simulink model "HANcoder_E407_TTA_Group2_REMOTE_72"  (R2018b)
settings: Solver=FixedStepDiscrete  StartTime=0.0  StopTime=1  FixedStep=0.01  RelTol=1e-3
PreLoadFcn:
  | librarySetup
  | eval([bdroot,'_startup']) %Calling [modelName]_startup.m
values from neighbouring files (symbols this model uses):
  BackUp_Role = 4    [HANcoder_E407_TTA_Group2_startup.m]
  basic_cycle_duration_bc0 = TM_Reset_Board   + COMP_duration    (= 320)    [HANcoder_E407_TTA_Group2_startup.m]    (also in HANcoder_E407_TTA_Template_startup.m = 212)
  basic_cycle_duration_bc1 = basic_cycle_duration_bc0    (= 320)    [HANcoder_E407_TTA_Group2_startup.m]    (also in HANcoder_E407_TTA_Template_startup.m = 212)
  board1_online = Simulink.Parameter    [HANcoder_E407_TTA_Group2_startup.m]
  board2_online = Simulink.Parameter    [HANcoder_E407_TTA_Group2_startup.m]
  board3_online = Simulink.Parameter    [HANcoder_E407_TTA_Group2_startup.m]
  board4_online = Simulink.Parameter    [HANcoder_E407_TTA_Group2_startup.m]
  comm_delay_estimation1 = round(comm_delay_measured1*hardware_granularity/frequency_IRQ)    [HANcoder_E407_TTA_Group2_startup.m]    (also in HANcoder_E407_TTA_Template_startup.m)
  comm_delay_estimation2 = round(comm_delay_measured2*hardware_granularity/frequency_IRQ)    [HANcoder_E407_TTA_Group2_startup.m]    (also in HANcoder_E407_TTA_Template_startup.m)
  COMM_Period = 40    [HANcoder_E407_TTA_Group2_startup.m]    (also in HANcoder_E407_TTA_Template_startup.m)
  COMM_Phase1 = Simulink.Parameter    [HANcoder_E407_TTA_Group2_startup.m]    (also in HANcoder_E407_TTA_Template_startup.m)
  COMM_Phase2 = Simulink.Parameter    [HANcoder_E407_TTA_Group2_startup.m]    (also in HANcoder_E407_TTA_Template_startup.m)
  COMM_Phase_init1 = Simulink.Parameter    [HANcoder_E407_TTA_Group2_startup.m]    (also in HANcoder_E407_TTA_Template_startup.m)
  COMM_Phase_init2 = Simulink.Parameter    [HANcoder_E407_TTA_Group2_startup.m]    (also in HANcoder_E407_TTA_Template_startup.m)
  COMP_duration = 8    [HANcoder_E407_TTA_Group2_startup.m]    (also in HANcoder_E407_TTA_Template_startup.m = 4)
  Controller1_Board = 1    [HANcoder_E407_TTA_Group2_startup.m]    (also in HANcoder_E407_TTA_Template_startup.m)
  Controller2_Board = 2    [HANcoder_E407_TTA_Group2_startup.m]    (also in HANcoder_E407_TTA_Template_startup.m)
  Controller3_Board = 3    [HANcoder_E407_TTA_Group2_startup.m]    (also in HANcoder_E407_TTA_Template_startup.m)
  Controller4_Board = 4    [HANcoder_E407_TTA_Group2_startup.m]
  delta_a_set = Simulink.Parameter    [HANcoder_E407_TTA_Group2_startup.m]
  delta_f_set = Simulink.Parameter    [HANcoder_E407_TTA_Group2_startup.m]
  delta_max = 1    [HANcoder_E407_TTA_Group2_startup.m]
  delta_min = -1    [HANcoder_E407_TTA_Group2_startup.m]
  delta_precision = 6    [HANcoder_E407_TTA_Group2_startup.m]
  frequency_IRQ = 100    [HANcoder_E407_TTA_Group2_startup.m]    (also in HANcoder_E407_TTA_Template_startup.m)
  HANtuneOverride = Simulink.Parameter    [HANcoder_E407_TTA_Group2_startup.m]    (also in HANcoder_E407_TTA_Template_startup.m)
  hardware_granularity = 1000000    [HANcoder_E407_TTA_Group2_startup.m]    (also in HANcoder_E407_TTA_Template_startup.m)
  I_a = 2.25    [HANcoder_E407_TTA_Group2_startup.m]
  I_f = 2.25    [HANcoder_E407_TTA_Group2_startup.m]
  idle_time_init = basic_cycle_duration_bc0 + basic_cycle_duration_bc1    (= 640)    [HANcoder_E407_TTA_Group2_startup.m]    (also in HANcoder_E407_TTA_Template_startup.m = 424)
  Input_Gen_Board = 5    [HANcoder_E407_TTA_Group2_startup.m]
  LA_Clock_Gr = 1    [HANcoder_E407_TTA_Group2_startup.m]    (also in HANcoder_E407_TTA_Template_startup.m)
  LA_COMM_dly = 1    [HANcoder_E407_TTA_Group2_startup.m]    (also in HANcoder_E407_TTA_Template_startup.m)
  LA_COMM_Err = 1    [HANcoder_E407_TTA_Group2_startup.m]    (also in HANcoder_E407_TTA_Template_startup.m)
  LA_E_Desync = 1    [HANcoder_E407_TTA_Group2_startup.m]    (also in HANcoder_E407_TTA_Template_startup.m)
  LA_MEX_Flag = 1    [HANcoder_E407_TTA_Group2_startup.m]    (also in HANcoder_E407_TTA_Template_startup.m)
  LA_Task_Act = 1    [HANcoder_E407_TTA_Group2_startup.m]    (also in HANcoder_E407_TTA_Template_startup.m)
  m_v = 100.0    (= 100)    [HANcoder_E407_TTA_Group2_startup.m]
  Master_Role = 1    [HANcoder_E407_TTA_Group2_startup.m]    (also in HANcoder_E407_TTA_Template_startup.m)
  matrix_cycle_duration = basic_cycle_duration_bc0 + basic_cycle_duration_bc1    (= 640)    [HANcoder_E407_TTA_Group2_startup.m]    (also in HANcoder_E407_TTA_Template_startup.m = 424)
  matrix_rows = 2    [HANcoder_E407_TTA_Group2_startup.m]    (also in HANcoder_E407_TTA_Template_startup.m)
  max_desync = 15    [HANcoder_E407_TTA_Group2_startup.m]    (also in HANcoder_E407_TTA_Template_startup.m)
  max_num_msgs_CAN1 = 2^Tx_bit_number-1    (= 7)    [HANcoder_E407_TTA_Group2_startup.m]    (also in HANcoder_E407_TTA_Template_startup.m)
  max_num_msgs_CAN2 = max_num_msgs_CAN1    (= 7)    [HANcoder_E407_TTA_Group2_startup.m]    (also in HANcoder_E407_TTA_Template_startup.m)
  min_desync = (-1)*max_desync    (= -15)    [HANcoder_E407_TTA_Group2_startup.m]    (also in HANcoder_E407_TTA_Template_startup.m)
  OutControl1_ID = 23    [HANcoder_E407_TTA_Group2_startup.m]    (also in HANcoder_E407_TTA_Template_startup.m)
  OutControl2_ID = 24    [HANcoder_E407_TTA_Group2_startup.m]    (also in HANcoder_E407_TTA_Template_startup.m)
  OutEmulator_ID = 25    [HANcoder_E407_TTA_Group2_startup.m]    (also in HANcoder_E407_TTA_Template_startup.m)
  R_al = 0.10    (= 0.1)    [HANcoder_E407_TTA_Group2_startup.m]
  R_ar = 0.10    (= 0.1)    [HANcoder_E407_TTA_Group2_startup.m]
  R_fl = 0.10    (= 0.1)    [HANcoder_E407_TTA_Group2_startup.m]
  R_fr = 0.10    (= 0.1)    [HANcoder_E407_TTA_Group2_startup.m]
  script_run = Simulink.Parameter    [HANcoder_E407_TTA_Group2_startup.m]    (also in HANcoder_E407_TTA_Template_startup.m)
  SensorValues_ID = 22    [HANcoder_E407_TTA_Group2_startup.m]    (also in HANcoder_E407_TTA_Template_startup.m)
  SetValues_ID = 21    [HANcoder_E407_TTA_Group2_startup.m]    (also in HANcoder_E407_TTA_Template_startup.m)
  Slave_Role = 3    [HANcoder_E407_TTA_Group2_startup.m]    (also in HANcoder_E407_TTA_Template_startup.m = 2)
  speed_max = 10    [HANcoder_E407_TTA_Group2_startup.m]
  speed_min = -10    [HANcoder_E407_TTA_Group2_startup.m]
  speed_precision = 3    [HANcoder_E407_TTA_Group2_startup.m]
  Sync_ID = 1    [HANcoder_E407_TTA_Group2_startup.m]    (also in HANcoder_E407_TTA_Template_startup.m)
  tau_max = 5    [HANcoder_E407_TTA_Group2_startup.m]
  tau_min = -5    [HANcoder_E407_TTA_Group2_startup.m]
  testV_1 = Simulink.Parameter    [HANcoder_E407_TTA_Group2_startup.m]
  testV_2 = Simulink.Parameter    [HANcoder_E407_TTA_Group2_startup.m]
  testV_3 = Simulink.Parameter    [HANcoder_E407_TTA_Group2_startup.m]
  theta_max = (speed_max/R_fr)*matrix_cycle_duration*frequency_IRQ/hardware_granularity    (= 6.4)    [HANcoder_E407_TTA_Group2_startup.m]
  theta_min = (-1)*theta_max    (= -6.4)    [HANcoder_E407_TTA_Group2_startup.m]
  theta_precision = 7-(fix(log2(theta_max))+1)    [HANcoder_E407_TTA_Group2_startup.m]
  Tl_a = 0.6    [HANcoder_E407_TTA_Group2_startup.m]
  Tl_f = 0.6    [HANcoder_E407_TTA_Group2_startup.m]
  TM_bc0_1 = basic_cycle_start    (= 0)    [HANcoder_E407_TTA_Group2_startup.m]
  TM_bc0_10 = TM_bc0_9 + COMP_duration    (= 168)    [HANcoder_E407_TTA_Group2_startup.m]
  TM_bc0_11 = TM_bc0_10 + COMP_duration    (= 176)    [HANcoder_E407_TTA_Group2_startup.m]
  TM_bc0_12 = TM_bc0_11  + COMM_duration    (= 216)    [HANcoder_E407_TTA_Group2_startup.m]
  TM_bc0_13 = TM_bc0_12 + COMP_duration    (= 224)    [HANcoder_E407_TTA_Group2_startup.m]
  TM_bc0_14 = TM_bc0_13 + COMP_duration    (= 232)    [HANcoder_E407_TTA_Group2_startup.m]
  TM_bc0_15 = TM_bc0_14  + COMM_duration    (= 272)    [HANcoder_E407_TTA_Group2_startup.m]
  TM_bc0_16 = TM_bc0_15 + COMP_duration    (= 280)    [HANcoder_E407_TTA_Group2_startup.m]
  TM_bc0_17 = TM_bc0_16 + COMP_duration    (= 288)    [HANcoder_E407_TTA_Group2_startup.m]
  TM_bc0_18 = TM_bc0_17 + COMP_duration    (= 296)    [HANcoder_E407_TTA_Group2_startup.m]
  TM_bc0_2 = TM_bc0_1   + COMM_duration    (= 40)    [HANcoder_E407_TTA_Group2_startup.m]
  TM_bc0_3 = TM_bc0_2  + COMP_duration    (= 48)    [HANcoder_E407_TTA_Group2_startup.m]
  TM_bc0_3_2 = TM_bc0_3   + 2    (= 50)    [HANcoder_E407_TTA_Group2_startup.m]
  TM_bc0_4 = TM_bc0_3   + COMP_duration    (= 56)    [HANcoder_E407_TTA_Group2_startup.m]
  TM_bc0_4_2 = TM_bc0_4    + 2    (= 58)    [HANcoder_E407_TTA_Group2_startup.m]
  TM_bc0_5 = TM_bc0_4    + COMP_duration    (= 64)    [HANcoder_E407_TTA_Group2_startup.m]
  TM_bc0_6 = TM_bc0_5  + COMM_duration    (= 104)    [HANcoder_E407_TTA_Group2_startup.m]
  TM_bc0_7 = TM_bc0_6 + COMP_duration    (= 112)    [HANcoder_E407_TTA_Group2_startup.m]
  TM_bc0_8 = TM_bc0_7 + COMP_duration    (= 120)    [HANcoder_E407_TTA_Group2_startup.m]
  TM_bc0_9 = TM_bc0_8  + COMM_duration    (= 160)    [HANcoder_E407_TTA_Group2_startup.m]
  TM_Check_Output_Control1 = TM_COMM_Output_Control1 + COMP_duration    (= 216)    [HANcoder_E407_TTA_Group2_startup.m]
  TM_Check_Sensor_Values = TM_COMM_Sensor_Values + COMM_duration    (= 144)    [HANcoder_E407_TTA_Group2_startup.m]
  TM_Check_Sensor_Values_2 = TM_Check_Sensor_Values + 2    (= 146)    [HANcoder_E407_TTA_Group2_startup.m]
  TM_Check_Set_Values = TM_COMM_Set_Values + COMM_duration    (= 96)    [HANcoder_E407_TTA_Group2_startup.m]
  TM_Check_Set_Values_2 = TM_Check_Set_Values + 2    (= 98)    [HANcoder_E407_TTA_Group2_startup.m]
  TM_Check_Sync = TM_COMM_Sync   + COMM_duration    (= 40)    [HANcoder_E407_TTA_Template_startup.m]
  TM_Check_Vote1 = TM_COMM_Vote1  + COMM_duration    (= 92)    [HANcoder_E407_TTA_Template_startup.m]
  TM_Check_Vote2 = TM_COMM_Vote2  + COMM_duration    (= 140)    [HANcoder_E407_TTA_Template_startup.m]
  TM_Check_Vote2_2 = TM_Check_Vote2 + 2    (= 142)    [HANcoder_E407_TTA_Template_startup.m]
  TM_COMM_Output_Control1 = TM_Velocity + COMM_duration    (= 208)    [HANcoder_E407_TTA_Group2_startup.m]
  TM_COMM_Output_Control1_2 = TM_COMM_Output_Control1 + 2    (= 210)    [HANcoder_E407_TTA_Group2_startup.m]
  TM_COMM_Sensor_Values = TM_Check_Set_Values + COMP_duration    (= 104)    [HANcoder_E407_TTA_Group2_startup.m]
  TM_COMM_Set_Values = TM_bc0_3 + COMP_duration    (= 56)    [HANcoder_E407_TTA_Group2_startup.m]
  TM_COMM_Sync = basic_cycle_start    (= 0)    [HANcoder_E407_TTA_Group2_startup.m]    (also in HANcoder_E407_TTA_Template_startup.m)
  TM_Count_Vote1 = TM_Check_Vote1 + COMP_duration    (= 96)    [HANcoder_E407_TTA_Template_startup.m]
  TM_Data_bc0 = TM_COMM_Sync    (= 0)    [HANcoder_E407_TTA_Group2_startup.m]    (also in HANcoder_E407_TTA_Template_startup.m)
  TM_Data_bc1 = TM_Data_bc0(1:4)    [HANcoder_E407_TTA_Group2_startup.m]    (also in HANcoder_E407_TTA_Template_startup.m)
  TM_Reset_Board = TM_Reset_Var   + COMP_duration    (= 312)    [HANcoder_E407_TTA_Group2_startup.m]    (also in HANcoder_E407_TTA_Template_startup.m = 208)
  TM_Reset_Var = TM_bc0_18  + COMP_duration    (= 304)    [HANcoder_E407_TTA_Group2_startup.m]    (also in HANcoder_E407_TTA_Template_startup.m = 204)
  TM_Reset_Var_bc1 = TM_bc0_14 + COMP_duration    (= 240)    [HANcoder_E407_TTA_Group2_startup.m]    (also in HANcoder_E407_TTA_Template_startup.m = 200)
  TM_Reset_Var_bc1_2 = TM_Reset_Var_bc1 + 2    (= 242)    [HANcoder_E407_TTA_Group2_startup.m]    (also in HANcoder_E407_TTA_Template_startup.m = 202)
  TM_Steer = TM_Check_Sensor_Values + COMP_duration    (= 152)    [HANcoder_E407_TTA_Group2_startup.m]
  TM_Torque = TM_Steer + COMP_duration    (= 160)    [HANcoder_E407_TTA_Group2_startup.m]
  TM_Type_bc0 = COMM    (= 0)    [HANcoder_E407_TTA_Group2_startup.m]    (also in HANcoder_E407_TTA_Template_startup.m)
  TM_Type_bc1 = TM_Type_bc0(1:4)    [HANcoder_E407_TTA_Group2_startup.m]    (also in HANcoder_E407_TTA_Template_startup.m)
  TM_Update_LT = TM_Check_Sync  + COMP_duration    (= 44)    [HANcoder_E407_TTA_Template_startup.m]
  TM_Update_LT_2 = TM_Update_LT   + 2    (= 46)    [HANcoder_E407_TTA_Template_startup.m]
  TM_Velocity = TM_Torque + COMP_duration    (= 168)    [HANcoder_E407_TTA_Group2_startup.m]
  TM_Vote_Dec = TM_Update_LT   + COMP_duration    (= 48)    [HANcoder_E407_TTA_Template_startup.m]
  torque_precision = 4    [HANcoder_E407_TTA_Group2_startup.m]
  ... (+7 more)
undefined symbols (not defined in the file or in its folder): A0, A1, A2, A3, A4, CON2, CON4, D10, D12, D13, D8, D9, TM_Check_Output_Emulator, TM_Check_Output_Emulator_2, TM_COMM_Output_Emulator
libraries: hdlsllib x247, HANcoder_STM32_Target x28, simulink x5, simulink_extras x1
(part 7 of 29)

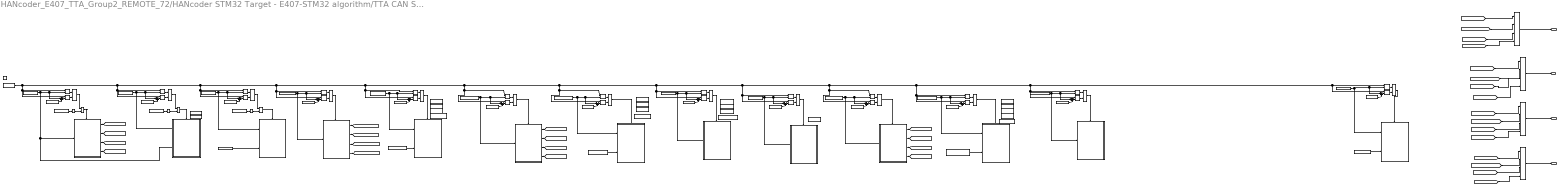
== system HANcoder_E407_TTA_Group2_REMOTE_72/HANcoder STM32 Target - E407-STM32 algorithm/TTA CAN System/TTA System/Matrix Cycle Manager/Controller Matrix Cycle/controller basic cycle 1 ==
  note: Output Send_Message
      | Send: 1
      | Do not send: 0
  note: Output Receive_Message
      | Receive: 1
      | Do not receive: 0
  note: Output Receive_Message
      | Receive: 1
      | Do not receive: 0
  note: Output Send_Message
      | Send: 1
      | Do not send: 0
  note: COMM - TW check
  note: COMP - TW check
  note: Local Time still not updated
  note: COMP - TW check
  note: Local Time still not updated
  note: Local Time still not updated
  note: COMP - TW check
  note: COMM - TW check
  note: COMP - TW check
  note: Send message condition
      | Sync Msg: Master and TM0
      | Vote Msg: Node# and TM#
  note: COMP - TW check
  note: COMP - TW check
  note: COMP - TW check
  note: COMM - TW check
  note: COMM - TW check
  note: COMP - TW check
  note: COMP - TW check
  Enable : EnablePort
  AND{,1..11,17..20} (16 alike) : Logic  IconShape=distinctive  AllPortsSameDT=off  OutDataTypeStr=boolean
  COMM Task - Set_Values : Subsystem
  COMM Task - Sync bc 1 : Subsystem
  COMM Task - Test1 : Subsystem
  COMM Task - send_BS : Subsystem
  "COMP Task - Do calculations " : Subsystem
  COMP Task - Get master Up to date : Subsystem
  COMP Task - Process_BS_Msg : Subsystem
  COMP Task - Reset Variables BC1 : Subsystem
  COMP Task - Rx_Set_Values_Check : Subsystem
  COMP Task - Sync bc1 check : Subsystem
  COMP Task - Test Receive1 : Subsystem
  COMP Task - Update LT1 : Subsystem
  COMP Task - Voting : Subsystem
  Constant : Constant  Value=TM_bc0_1
  Constant{1,10,18,21} (4 alike) : Constant  Value=COMM_Period
  Constant{2..3,9,11,15,20,22,27,29} (9 alike) : Constant  Value=COMP_duration
  Constant12 : Constant  Value=TM_COMM_Output_Control1
  Constant13 : Constant  Value=TM_COMM_Output_Control1_2
  Constant14 : Constant  Value=TM_Torque
  Constant16 : Constant  Value=TM_Reset_Var_bc1
  Constant17 : Constant  Value=TM_bc0_3_2
  Constant19 : Constant  Value=TM_Check_Set_Values_2
  Constant23 : Constant  Value=TM_Check_Sensor_Values
  Constant24 : Constant  Value=TM_Check_Sensor_Values_2
  Constant25 : Constant  Value=TM_COMM_Sensor_Values
  Constant26 : Constant  Value=TM_Check_Output_Control1
  Constant28 : Constant  Value=TM_Steer
  Constant4 : Constant  Value=TM_bc0_2
  Constant41 : Constant  Value=TM_Reset_Var_bc1_2
  Constant5 : Constant  Value=TM_COMM_Set_Values
  Constant6 : Constant  Value=TM_bc0_3
  Constant7 : Constant  Value=TM_Check_Set_Values
  Constant8 : Constant  Value=TM_Velocity
  Data Store Memory1 : DataStoreMemory  DataStoreName=Error_BS_NotRX  ReadBeforeWriteMsg=warning  WriteAfterWriteMsg=warning  WriteAfterReadMsg=warning  ShowAdditionalParam=off  OutDataTypeStr=boolean
  Data Store Memory10 : DataStoreMemory  DataStoreName=v_set_stored  ReadBeforeWriteMsg=warning  WriteAfterWriteMsg=warning  WriteAfterReadMsg=warning  ShowAdditionalParam=off
  Data Store Memory11 : DataStoreMemory  DataStoreName=Msg_Rx  ReadBeforeWriteMsg=warning  WriteAfterWriteMsg=warning  WriteAfterReadMsg=warning  ShowAdditionalParam=off  OutDataTypeStr=Bus: msg_buffer_type
  Data Store Memory12 : DataStoreMemory  DataStoreName=Error_SensorValues_NotRX  ReadBeforeWriteMsg=warning  WriteAfterWriteMsg=warning  WriteAfterReadMsg=warning  ShowAdditionalParam=off  OutDataTypeStr=boolean
  Data Store Memory13 : DataStoreMemory  DataStoreName=Error_Test_NotRX  ReadBeforeWriteMsg=warning  WriteAfterWriteMsg=warning  WriteAfterReadMsg=warning  ShowAdditionalParam=off  OutDataTypeStr=boolean
  Data Store Memory14 : DataStoreMemory  DataStoreName=rxTest3  ReadBeforeWriteMsg=warning  WriteAfterWriteMsg=warning  WriteAfterReadMsg=warning  ShowAdditionalParam=off
  Data Store Memory15 : DataStoreMemory  DataStoreName=rxTest1  ReadBeforeWriteMsg=warning  WriteAfterWriteMsg=warning  WriteAfterReadMsg=warning  ShowAdditionalParam=off
  Data Store Memory16 : DataStoreMemory  DataStoreName=rxTest2  ReadBeforeWriteMsg=warning  WriteAfterWriteMsg=warning  WriteAfterReadMsg=warning  ShowAdditionalParam=off
  Data Store Memory17 : DataStoreMemory  DataStoreName=B2  ReadBeforeWriteMsg=warning  WriteAfterWriteMsg=warning  WriteAfterReadMsg=warning  ShowAdditionalParam=off
  Data Store Memory2 : DataStoreMemory  DataStoreName=B4  ReadBeforeWriteMsg=warning  WriteAfterWriteMsg=warning  WriteAfterReadMsg=warning  ShowAdditionalParam=off
  Data Store Memory20 : DataStoreMemory  DataStoreName=delta_f_set_stored  ReadBeforeWriteMsg=warning  WriteAfterWriteMsg=warning  WriteAfterReadMsg=warning  ShowAdditionalParam=off
  Data Store Memory28 : DataStoreMemory  DataStoreName=Error_SetValues_NotRX  ReadBeforeWriteMsg=warning  WriteAfterWriteMsg=warning  WriteAfterReadMsg=warning  ShowAdditionalParam=off  OutDataTypeStr=boolean
  Data Store Memory3 : DataStoreMemory  DataStoreName=B3  ReadBeforeWriteMsg=warning  WriteAfterWriteMsg=warning  WriteAfterReadMsg=warning  ShowAdditionalParam=off
  Data Store Memory31 : DataStoreMemory  DataStoreName=delta_a_set_stored  ReadBeforeWriteMsg=warning  WriteAfterWriteMsg=warning  WriteAfterReadMsg=warning  ShowAdditionalParam=off
  Data Store Memory4 : DataStoreMemory  DataStoreName=B1  ReadBeforeWriteMsg=warning  WriteAfterWriteMsg=warning  WriteAfterReadMsg=warning  ShowAdditionalParam=off
  Data Store Memory5 : DataStoreMemory  DataStoreName=Test3  ReadBeforeWriteMsg=warning  WriteAfterWriteMsg=warning  WriteAfterReadMsg=warning  ShowAdditionalParam=off
  Data Store Memory6 : DataStoreMemory  DataStoreName=Test1  ReadBeforeWriteMsg=warning  WriteAfterWriteMsg=warning  WriteAfterReadMsg=warning  ShowAdditionalParam=off
  Data Store Memory7 : DataStoreMemory  DataStoreName=Test2  ReadBeforeWriteMsg=warning  WriteAfterWriteMsg=warning  WriteAfterReadMsg=warning  ShowAdditionalParam=off
  Data Store Memory8 : DataStoreMemory  DataStoreName=new_msg_Rx  ReadBeforeWriteMsg=warning  WriteAfterWriteMsg=warning  WriteAfterReadMsg=warning  ShowAdditionalParam=off
  Data Store Memory9 : DataStoreMemory  DataStoreName=votingOut  ReadBeforeWriteMsg=warning  WriteAfterWriteMsg=warning  WriteAfterReadMsg=warning  ShowAdditionalParam=off
  Data Store Read1 : DataStoreRead  DataStoreName=Local_Ticks
  Data Store Read11 : DataStoreRead  DataStoreName=BC1_Sync_processed
  Data Store Read6 : DataStoreRead  DataStoreName=BC1_Sync_processed
  Data Store Read7 : DataStoreRead  DataStoreName=BC1_Sync_processed
  GreaterThan{,2,4,6,8,10,12,14,16,18,20,22,34} (13 alike) : RelationalOperator  OutDataTypeStr=boolean  RndMeth=Simplest
  GreaterThan{1,3,5,7,9,11,13,15,17,19,21,23,35} (13 alike) : RelationalOperator  Operator=<  OutDataTypeStr=boolean  RndMeth=Simplest
  NOT2 : Logic  Operator=NOT  IconShape=distinctive  AllPortsSameDT=off  OutDataTypeStr=boolean
  NOT4 : Logic  Operator=NOT  IconShape=distinctive  AllPortsSameDT=off  OutDataTypeStr=boolean
  NOT5 : Logic  Operator=NOT  IconShape=distinctive  AllPortsSameDT=off  OutDataTypeStr=boolean
  OR{1..4} (4 alike) : Logic  Operator=OR  Inputs=4  IconShape=distinctive  AllPortsSameDT=off  OutDataTypeStr=boolean
  Sum{1..12,18} (13 alike) : Sum  Inputs=|++
  Send_Message_CAN1 : Outport  OutputWhenDisabled=reset  InitialOutput=0
  Send_Message_CAN2 : Outport  Port=2  OutputWhenDisabled=reset  InitialOutput=0
  Receive_Message_CAN1 : Outport  Port=3  OutputWhenDisabled=reset  InitialOutput=0
  Receive_Message_CAN2 : Outport  Port=4  OutputWhenDisabled=reset  InitialOutput=0
  wires:
  Constant1/1 -> Sum4/2
  COMM Task - Sync bc 1/1(Send CAN1) -> [send_CAN1_Sync_bc1_TAG]
  COMM Task - Sync bc 1/2(Receive CAN1) -> [receive_CAN1_Sync_bc1_TAG]
  COMM Task - Sync bc 1/4(Receive CAN2) -> [receive_CAN2_Sync_bc1_TAG]
  AND19/1 -> COMP Task - Update LT1/Enable
  NOT2/1 -> AND18/2
  Data Store Read7/1 -> NOT5/1
  GreaterThan4/1 -> AND2/1
  AND18/1 -> COMP Task - Sync bc1 check/Enable
  AND1/1 -> AND18/1
  Data Store Read11/1 -> NOT4/1
  AND17/1 -> COMM Task - Sync bc 1/Enable
  AND2/1 -> AND19/1
  Data Store Read6/1 -> NOT2/1
  NOT4/1 -> AND17/2
  GreaterThan1/1 -> AND/2
  GreaterThan/1 -> AND/1
  Constant/1 -> COMP Task - Sync bc1 check/2(TM_COMM), COMM Task - Sync bc 1/1(Time Mark), Sum4/1, GreaterThan/2
  AND/1 -> AND17/1
  Constant3/1 -> Sum2/2
  Constant6/1 -> COMP Task - Update LT1/1(Time_Mark), Sum2/1, GreaterThan4/2
  Sum4/1 -> GreaterThan1/2
  GreaterThan2/1 -> AND1/1
  GreaterThan3/1 -> AND1/2
  Constant2/1 -> Sum1/2
  Constant4/1 -> COMP Task - Sync bc1 check/1(Time_Mark), GreaterThan2/2, Sum1/1
  Sum1/1 -> GreaterThan3/2
  COMM Task - Sync bc 1/3(Send CAN2) -> [send_CAN2_Sync_bc1_TAG]
  NOT5/1 -> AND19/2
  Sum2/1 -> GreaterThan5/2
  GreaterThan5/1 -> AND2/2
  GreaterThan35/1 -> AND20/2
  Constant16/1 -> Sum18/1, GreaterThan34/2, COMP Task - Reset Variables BC1/1(Time_Mark)
  Constant15/1 -> Sum18/2
  Sum18/1 -> GreaterThan35/2
  GreaterThan34/1 -> AND20/1
  AND20/1 -> COMP Task - Reset Variables BC1/Enable
  Constant17/1 -> COMP Task - Update LT1/2(Time_Mark_2)
  Constant41/1 -> COMP Task - Reset Variables BC1/2(Time_Mark_2)
  GreaterThan7/1 -> AND3/2
  COMM Task - Set_Values/2(Receive CAN1) -> [receive_CAN1_Set_Values_bc1_TAG]
  Sum5/1 -> GreaterThan9/2
  COMM Task - Set_Values/4(Receive CAN2) -> [receive_CAN2_Set_Values_bc1_TAG]
  COMM Task - Set_Values/3(Send CAN2) -> [send_CAN2_Set_Values_bc1_TAG]
  GreaterThan6/1 -> AND3/1
  COMM Task - Set_Values/1(Send CAN1) -> [send_CAN1_Set_Values_bc1_TAG]
  Constant19/1 -> COMP Task - Rx_Set_Values_Check/2(Time_Mark_2)
  GreaterThan9/1 -> AND4/2
  AND4/1 -> COMP Task - Rx_Set_Values_Check/Enable
  GreaterThan8/1 -> AND4/1
  Constant9/1 -> Sum5/2
  Sum3/1 -> GreaterThan7/2
  Constant7/1 -> COMP Task - Rx_Set_Values_Check/1(Time_Mark), Sum5/1, GreaterThan8/2
  Constant18/1 -> Sum3/2
  Constant5/1 -> COMM Task - Set_Values/1(Time Mark), GreaterThan6/2, Sum3/1
  AND3/1 -> COMM Task - Set_Values/Enable
  OR1/1 -> Send_Message_CAN1/1
  [send_CAN1_Set_Values_bc1_TAG] -> OR1/2
  [send_CAN1_Sync_bc1_TAG] -> OR1/1
  [receive_CAN2_Sync_bc1_TAG] -> OR4/1
  [receive_CAN1_Sync_bc1_TAG] -> OR3/1
  [send_CAN2_Sync_bc1_TAG] -> OR2/1
  OR3/1 -> Receive_Message_CAN1/1
  OR4/1 -> Receive_Message_CAN2/1
  [send_CAN2_Set_Values_bc1_TAG] -> OR2/2
  [receive_CAN1_Set_Values_bc1_TAG] -> OR3/2
  [receive_CAN2_Set_Values_bc1_TAG] -> OR4/2
  OR2/1 -> Send_Message_CAN2/1
  [receive_CAN2_Test_bc1_TAG] -> OR4/3
  [receive_CAN1_Test_bc1_TAG] -> OR3/3
  [send_CAN2_Test_bc1_TAG] -> OR2/3
  [send_CAN1_Test_bc1_TAG] -> OR1/3
  Constant29/1 -> Sum8/2
  Sum8/1 -> GreaterThan19/2
  GreaterThan18/1 -> AND7/1
  GreaterThan19/1 -> AND7/2
  AND7/1 -> "COMP Task - Do calculations "/Enable
  Constant28/1 -> "COMP Task - Do calculations "/1(Time_Mark), GreaterThan18/2, Sum8/1
  Constant14/1 -> COMP Task - Voting/1(Time_Mark), GreaterThan14/2, Sum9/1
  GreaterThan15/1 -> AND8/2
  Constant20/1 -> Sum9/2
  AND8/1 -> COMP Task - Voting/Enable
  GreaterThan14/1 -> AND8/1
  Sum9/1 -> GreaterThan15/2
  GreaterThan17/1 -> AND9/2
  AND10/1 -> COMP Task - Test Receive1/Enable
  COMM Task - Test1/3(Send CAN2) -> [send_CAN2_Test_bc1_TAG]
  GreaterThan21/1 -> AND10/2
  Constant22/1 -> Sum10/2
  Constant25/1 -> COMM Task - Test1/1(Time Mark), Sum11/1, GreaterThan16/2
  GreaterThan16/1 -> AND9/1
  Constant21/1 -> Sum11/2
  Sum11/1 -> GreaterThan17/2
  AND9/1 -> COMM Task - Test1/Enable
  Sum10/1 -> GreaterThan21/2
  COMM Task - Test1/4(Receive CAN2) -> [receive_CAN2_Test_bc1_TAG]
  Constant23/1 -> COMP Task - Test Receive1/1(Time_Mark), GreaterThan20/2, Sum10/1
  GreaterThan20/1 -> AND10/1
  Constant24/1 -> COMP Task - Test Receive1/2(Time_Mark_2)
  COMM Task - Test1/2(Receive CAN1) -> [receive_CAN1_Test_bc1_TAG]
  COMM Task - Test1/1(Send CAN1) -> [send_CAN1_Test_bc1_TAG]
  Constant11/1 -> Sum6/2
  Sum7/1 -> GreaterThan11/2
  Constant13/1 -> COMP Task - Process_BS_Msg/2(Time_Mark_2)
  Constant10/1 -> Sum7/2
  AND5/1 -> COMM Task - send_BS/Enable
  Constant8/1 -> COMM Task - send_BS/1(Time Mark), Sum7/1, GreaterThan10/2
  Constant12/1 -> COMP Task - Process_BS_Msg/1(Time_Mark), GreaterThan12/2, Sum6/1
  COMM Task - send_BS/4(Receive CAN2) -> [receive_CAN2_BS_bc1_TAG]
  Sum6/1 -> GreaterThan13/2
  GreaterThan12/1 -> AND6/1
  COMM Task - send_BS/2(Receive CAN1) -> [receive_CAN1_BS_bc1_TAG]
  COMM Task - send_BS/1(Send CAN1) -> [send_CAN1_BS_bc1_TAG]
  GreaterThan13/1 -> AND6/2
  AND6/1 -> COMP Task - Process_BS_Msg/Enable
  GreaterThan11/1 -> AND5/2
  COMM Task - send_BS/3(Send CAN2) -> [send_CAN2_BS_bc1_TAG]
  GreaterThan10/1 -> AND5/1
  [send_CAN1_BS_bc1_TAG] -> OR1/4
  [send_CAN2_BS_bc1_TAG] -> OR2/4
  [receive_CAN2_BS_bc1_TAG] -> OR4/4
  [receive_CAN1_BS_bc1_TAG] -> OR3/4
  Constant27/1 -> Sum12/2
  GreaterThan22/1 -> AND11/1
  Constant26/1 -> COMP Task - Get master Up to date/1(Time_Mark), GreaterThan22/2, Sum12/1
  Sum12/1 -> GreaterThan23/2
  AND11/1 -> COMP Task - Get master Up to date/Enable
  GreaterThan23/1 -> AND11/2
  Data Store Read1/1 -> GreaterThan7/1, GreaterThan6/1, GreaterThan17/1, GreaterThan16/1, GreaterThan21/1, GreaterThan20/1, GreaterThan14/1, GreaterThan15/1, GreaterThan11/1, GreaterThan10/1, GreaterThan12/1, GreaterThan13/1, GreaterThan22/1, GreaterThan23/1, GreaterThan34/1, GreaterThan35/1, GreaterThan18/1, GreaterThan19/1, GreaterThan8/1, GreaterThan9/1, GreaterThan4/1, GreaterThan5/1, GreaterThan2/1, GreaterThan3/1, GreaterThan/1, GreaterThan1/1

== system HANcoder_E407_TTA_Group2_REMOTE_72/HANcoder STM32 Target - E407-STM32 algorithm/TTA CAN System/TTA System/Matrix Cycle Manager/Controller Matrix Cycle/msg_count_DEBUG observer ==
  Data Store Read24 : DataStoreRead  DataStoreName=msg_count_DEBUG
  Terminator : Terminator
  wires:
  Data Store Read24/1 -> Terminator/1  "msg_count_DEBUG_s"

== system HANcoder_E407_TTA_Group2_REMOTE_72/HANcoder STM32 Target - E407-STM32 algorithm/TTA CAN System/TTA System/Matrix Cycle Manager/Input Generator Matrix Cycle/Matrix_Cycle_Observation_DEBUG ==
  Data Store Read : DataStoreRead  DataStoreName=Master_ID
  Data Store Read1 : DataStoreRead  DataStoreName=Role_ID
  Data Store Read10 : DataStoreRead  DataStoreName=BC1_Sync_processed
  Data Store Read2 : DataStoreRead  DataStoreName=BC0_Sync_processed
  Data Store Read3 : DataStoreRead  DataStoreName=Sync_bc1_missed_counter
  Data Store Read4 : DataStoreRead  DataStoreName=Sync_bc0_missed_counter
  Terminator{,1..4,12} (6 alike) : Terminator
  wires:
  Data Store Read1/1 -> Terminator/1  "Role_ID_ing_s"
  Data Store Read10/1 -> Terminator12/1  "BC1_sync_processed_ing_s"
  Data Store Read2/1 -> Terminator2/1  "BC0_sync_processed_ing_s"
  Data Store Read/1 -> Terminator1/1  "Master_ID_ing_s"
  Data Store Read3/1 -> Terminator4/1  "sync_bc1_miss_counter_ing"
  Data Store Read4/1 -> Terminator3/1  "sync_bc0_miss_counter_ing"

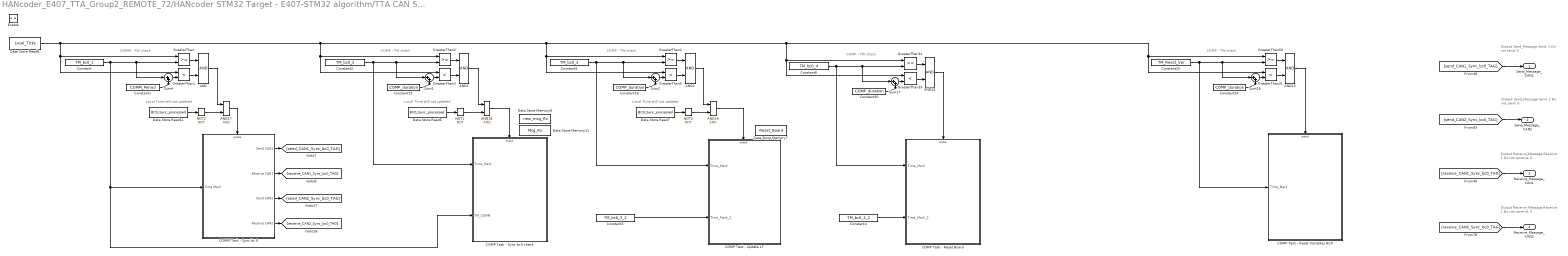
== system HANcoder_E407_TTA_Group2_REMOTE_72/HANcoder STM32 Target - E407-STM32 algorithm/TTA CAN System/TTA System/Matrix Cycle Manager/Input Generator Matrix Cycle/input generator basic cycle 0 ==
  note: Local Time still not updated
  note: Local Time still not updated
  note: Local Time still not updated
  note: COMP - TW check
  note: COMP - TW check
  note: COMP - TW check
  note: COMP - TW check
  note: COMM - TW check
  note: Output Receive_Message
      | Receive: 1
      | Do not receive: 0
  note: Output Send_Message
      | Send: 1
      | Do not send: 0
  note: Output Receive_Message
      | Receive: 1
      | Do not receive: 0
  note: Output Send_Message
      | Send: 1
      | Do not send: 0
  Enable : EnablePort  PropagateVarSize=During execution
  AND{,1..2,15..19} (8 alike) : Logic  IconShape=distinctive  AllPortsSameDT=off  OutDataTypeStr=boolean
  COMM Task - Sync bc 0 : Subsystem
  COMP Task - Reset Board : Subsystem
  COMP Task - Reset Variables BC0 : Subsystem
  COMP Task - Sync bc0 check : Subsystem
  COMP Task - Update LT : Subsystem
  Constant : Constant  Value=TM_bc0_1
  Constant1 : Constant  Value=COMM_Period
  Constant{15..16,24,30} (4 alike) : Constant  Value=COMP_duration
  Constant2 : Constant  Value=TM_bc0_2
  Constant25 : Constant  Value=TM_Reset_Var
  Constant3 : Constant  Value=TM_bc0_3_2
  Constant4 : Constant  Value=TM_bc0_4_2
  Constant5 : Constant  Value=TM_bc0_3
  Constant6 : Constant  Value=TM_bc0_4
  Data Store Memory11 : DataStoreMemory  DataStoreName=Msg_Rx  ReadBeforeWriteMsg=warning  WriteAfterWriteMsg=warning  WriteAfterReadMsg=warning  ShowAdditionalParam=off  OutDataTypeStr=Bus: msg_buffer_type
  Data Store Memory7 : DataStoreMemory  DataStoreName=Reset_Board  ReadBeforeWriteMsg=warning  WriteAfterWriteMsg=warning  WriteAfterReadMsg=warning  ShowAdditionalParam=off  OutDataTypeStr=boolean
  Data Store Memory8 : DataStoreMemory  DataStoreName=new_msg_Rx  ReadBeforeWriteMsg=warning  WriteAfterWriteMsg=warning  WriteAfterReadMsg=warning  ShowAdditionalParam=off
  Data Store Read11 : DataStoreRead  DataStoreName=BC0_Sync_processed
  Data Store Read6 : DataStoreRead  DataStoreName=BC0_Sync_processed
  Data Store Read7 : DataStoreRead  DataStoreName=BC0_Sync_processed
  Data Store Read8 : DataStoreRead  DataStoreName=Local_Ticks
  GreaterThan{,2,4,30,32} (5 alike) : RelationalOperator  OutDataTypeStr=boolean  RndMeth=Simplest
  GreaterThan{1,3,5,31,33} (5 alike) : RelationalOperator  Operator=<  OutDataTypeStr=boolean  RndMeth=Simplest
  NOT1 : Logic  Operator=NOT  IconShape=distinctive  AllPortsSameDT=off  OutDataTypeStr=boolean
  NOT2 : Logic  Operator=NOT  IconShape=distinctive  AllPortsSameDT=off  OutDataTypeStr=boolean
  NOT3 : Logic  Operator=NOT  IconShape=distinctive  AllPortsSameDT=off  OutDataTypeStr=boolean
  Sum{1..2,4,16..17} (5 alike) : Sum  Inputs=|++
  Send_Message_CAN1 : Outport  OutputWhenDisabled=reset  InitialOutput=0
  Send_Message_CAN2 : Outport  Port=2  OutputWhenDisabled=reset  InitialOutput=0
  Receive_Message_CAN1 : Outport  Port=3  OutputWhenDisabled=reset  InitialOutput=0
  Receive_Message_CAN2 : Outport  Port=4  OutputWhenDisabled=reset  InitialOutput=0
  wires:
  AND19/1 -> COMP Task - Update LT/Enable
  AND2/1 -> AND19/1
  NOT3/1 -> AND19/2
  Data Store Read7/1 -> NOT3/1
  AND18/1 -> COMP Task - Sync bc0 check/Enable
  AND1/1 -> AND18/1
  NOT1/1 -> AND18/2
  Data Store Read6/1 -> NOT1/1
  AND17/1 -> COMM Task - Sync bc 0/Enable
  NOT2/1 -> AND17/2
  Data Store Read11/1 -> NOT2/1
  GreaterThan33/1 -> AND16/2
  Sum17/1 -> GreaterThan33/2
  GreaterThan32/1 -> AND16/1
  Constant30/1 -> Sum17/2
  Constant6/1 -> GreaterThan32/2, Sum17/1, COMP Task - Reset Board/1(Time_Mark)
  AND16/1 -> COMP Task - Reset Board/Enable
  Data Store Read8/1 -> GreaterThan1/1, GreaterThan/1, GreaterThan3/1, GreaterThan2/1, GreaterThan5/1, GreaterThan4/1, GreaterThan30/1, GreaterThan31/1, GreaterThan33/1, GreaterThan32/1
  AND15/1 -> COMP Task - Reset Variables BC0/Enable
  Constant25/1 -> Sum16/1, GreaterThan30/2, COMP Task - Reset Variables BC0/1(Time_Mark)
  Constant24/1 -> Sum16/2
  GreaterThan30/1 -> AND15/1
  Sum16/1 -> GreaterThan31/2
  GreaterThan31/1 -> AND15/2
  GreaterThan5/1 -> AND2/2
  GreaterThan4/1 -> AND2/1
  Sum2/1 -> GreaterThan5/2
  Constant5/1 -> GreaterThan4/2, Sum2/1, COMP Task - Update LT/1(Time_Mark)
  Constant16/1 -> Sum2/2
  Constant15/1 -> Sum1/2
  Constant2/1 -> Sum1/1, GreaterThan2/2, COMP Task - Sync bc0 check/1(Time_Mark)
  Sum1/1 -> GreaterThan3/2
  GreaterThan2/1 -> AND1/1
  GreaterThan3/1 -> AND1/2
  AND/1 -> AND17/1
  GreaterThan1/1 -> AND/2
  GreaterThan/1 -> AND/1
  Sum4/1 -> GreaterThan1/2
  Constant/1 -> GreaterThan/2, Sum4/1, COMM Task - Sync bc 0/1(Time Mark), COMP Task - Sync bc0 check/2(TM_COMM)
  Constant1/1 -> Sum4/2
  COMM Task - Sync bc 0/4(Receive CAN2) -> [receive_CAN2_Sync_bc0_TAG]
  COMM Task - Sync bc 0/3(Send CAN2) -> [send_CAN2_Sync_bc0_TAG]
  COMM Task - Sync bc 0/2(Receive CAN1) -> [receive_CAN1_Sync_bc0_TAG]
  COMM Task - Sync bc 0/1(Send CAN1) -> [send_CAN1_Sync_bc0_TAG]
  [send_CAN1_Sync_bc0_TAG] -> Send_Message_CAN1/1
  [send_CAN2_Sync_bc0_TAG] -> Send_Message_CAN2/1
  [receive_CAN1_Sync_bc0_TAG] -> Receive_Message_CAN1/1
  [receive_CAN2_Sync_bc0_TAG] -> Receive_Message_CAN2/1
  Constant3/1 -> COMP Task - Update LT/2(Time_Mark_2)
  Constant4/1 -> COMP Task - Reset Board/2(Time_Mark_2)

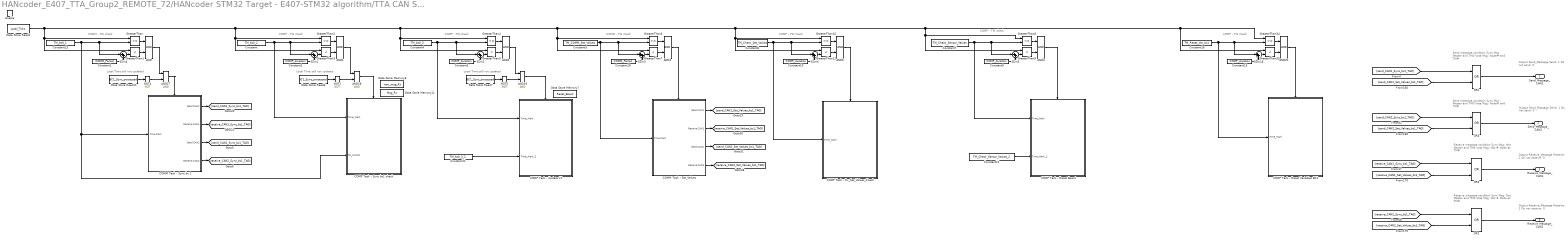
== system HANcoder_E407_TTA_Group2_REMOTE_72/HANcoder STM32 Target - E407-STM32 algorithm/TTA CAN System/TTA System/Matrix Cycle Manager/Input Generator Matrix Cycle/input generator basic cycle 1 ==
  note: COMP - TW check
  note: COMM - TW check
  note: Local Time still not updated
  note: Local Time still not updated
  note: COMP - TW check
  note: Local Time still not updated
  note: COMP - TW check
  note: COMP - TW check
  note: COMM - TW check
  note: Receive message condition
      | Sync Msg: Not Master and TM0
      | Vote Msg: Not # Node at TM#
  note: Send message condition
      | Sync Msg: Master and TM0
      | Vote Msg: Node# and TM#
  note: Output Send_Message
      | Send: 1
      | Do not send: 0
  note: Output Receive_Message
      | Receive: 1
      | Do not receive: 0
  note: Output Receive_Message
      | Receive: 1
      | Do not receive: 0
  note: Output Send_Message
      | Send: 1
      | Do not send: 0
  note: Send message condition
      | Sync Msg: Master and TM0
      | Vote Msg: Node# and TM#
  note: Receive message condition
      | Sync Msg: Not Master and TM0
      | Vote Msg: Not # Node at TM#
  note: COMP - TW check
  Enable : EnablePort
  AND{,1..5,17..20} (10 alike) : Logic  IconShape=distinctive  AllPortsSameDT=off  OutDataTypeStr=boolean
  COMM Task - Set_Values : Subsystem
  COMM Task - Sync bc 1 : Subsystem
  COMP Task - Reset Board : Subsystem
  COMP Task - Reset Variables BC1 : Subsystem
  COMP Task - Rx_Set_Values_Check : Subsystem
  COMP Task - Sync bc1 check : Subsystem
  COMP Task - Update LT : Subsystem
  Constant : Constant  Value=TM_bc0_2
  Constant1 : Constant  Value=COMM_Period
  Constant{2..3,9..10,15} (5 alike) : Constant  Value=COMP_duration
  Constant11 : Constant  Value=TM_bc0_3_2
  Constant12 : Constant  Value=TM_Check_Sensor_Values_2
  Constant13 : Constant  Value=TM_bc0_1
  Constant16 : Constant  Value=TM_Reset_Var_bc1
  Constant18 : Constant  Value=COMM_Period
  Constant4 : Constant  Value=TM_bc0_3
  Constant5 : Constant  Value=TM_COMM_Set_Values
  Constant7 : Constant  Value=TM_Check_Sensor_Values
  Constant8 : Constant  Value=TM_Check_Set_Values
  Data Store Memory11 : DataStoreMemory  DataStoreName=Msg_Rx  ReadBeforeWriteMsg=warning  WriteAfterWriteMsg=warning  WriteAfterReadMsg=warning  ShowAdditionalParam=off  OutDataTypeStr=Bus: msg_buffer_type
  Data Store Memory7 : DataStoreMemory  DataStoreName=Reset_Board  ReadBeforeWriteMsg=warning  WriteAfterWriteMsg=warning  WriteAfterReadMsg=warning  ShowAdditionalParam=off  OutDataTypeStr=boolean
  Data Store Memory8 : DataStoreMemory  DataStoreName=new_msg_Rx  ReadBeforeWriteMsg=warning  WriteAfterWriteMsg=warning  WriteAfterReadMsg=warning  ShowAdditionalParam=off
  Data Store Read1 : DataStoreRead  DataStoreName=Local_Ticks
  Data Store Read11 : DataStoreRead  DataStoreName=BC1_Sync_processed
  Data Store Read6 : DataStoreRead  DataStoreName=BC1_Sync_processed
  Data Store Read7 : DataStoreRead  DataStoreName=BC1_Sync_processed
  GreaterThan{,2,4,6,8,10,34} (7 alike) : RelationalOperator  OutDataTypeStr=boolean  RndMeth=Simplest
  GreaterThan{1,3,5,7,9,11,35} (7 alike) : RelationalOperator  Operator=<  OutDataTypeStr=boolean  RndMeth=Simplest
  NOT2 : Logic  Operator=NOT  IconShape=distinctive  AllPortsSameDT=off  OutDataTypeStr=boolean
  NOT4 : Logic  Operator=NOT  IconShape=distinctive  AllPortsSameDT=off  OutDataTypeStr=boolean
  NOT5 : Logic  Operator=NOT  IconShape=distinctive  AllPortsSameDT=off  OutDataTypeStr=boolean
  OR{1..4} (4 alike) : Logic  Operator=OR  IconShape=distinctive  AllPortsSameDT=off  OutDataTypeStr=boolean
  Sum{1..6,18} (7 alike) : Sum  Inputs=|++
  Send_Message_CAN1 : Outport  OutputWhenDisabled=reset  InitialOutput=0
  Send_Message_CAN2 : Outport  Port=2  OutputWhenDisabled=reset  InitialOutput=0
  Receive_Message_CAN1 : Outport  Port=3  OutputWhenDisabled=reset  InitialOutput=0
  Receive_Message_CAN2 : Outport  Port=4  OutputWhenDisabled=reset  InitialOutput=0
  wires:
  AND20/1 -> COMP Task - Reset Variables BC1/Enable
  GreaterThan34/1 -> AND20/1
  Sum18/1 -> GreaterThan35/2
  Constant15/1 -> Sum18/2
  Constant16/1 -> COMP Task - Reset Variables BC1/1(Time_Mark), GreaterThan34/2, Sum18/1
  GreaterThan35/1 -> AND20/2
  COMM Task - Set_Values/4(Receive CAN2) -> [receive_CAN2_Set_Values_bc1_TAG]
  COMM Task - Set_Values/3(Send CAN2) -> [send_CAN2_Set_Values_bc1_TAG]
  COMM Task - Set_Values/2(Receive CAN1) -> [receive_CAN1_Set_Values_bc1_TAG]
  COMM Task - Set_Values/1(Send CAN1) -> [send_CAN1_Set_Values_bc1_TAG]
  GreaterThan5/1 -> AND2/2
  Sum2/1 -> GreaterThan5/2
  NOT5/1 -> AND19/2
  COMM Task - Sync bc 1/3(Send CAN2) -> [send_CAN2_Sync_bc1_TAG]
  Sum1/1 -> GreaterThan3/2
  Constant/1 -> Sum1/1, GreaterThan2/2, COMP Task - Sync bc1 check/1(Time_Mark)
  GreaterThan7/1 -> AND3/2
  Constant2/1 -> Sum1/2
  GreaterThan3/1 -> AND1/2
  GreaterThan2/1 -> AND1/1
  GreaterThan9/1 -> AND4/2
  GreaterThan8/1 -> AND4/1
  GreaterThan6/1 -> AND3/1
  Sum4/1 -> GreaterThan1/2
  Sum5/1 -> GreaterThan9/2
  Constant4/1 -> COMP Task - Update LT/1(Time_Mark), GreaterThan4/2, Sum2/1
  Sum3/1 -> GreaterThan7/2
  Constant7/1 -> COMP Task - Reset Board/1(Time_Mark), GreaterThan8/2, Sum5/1
  Constant3/1 -> Sum2/2
  AND/1 -> AND17/1
  Constant18/1 -> Sum3/2
  Constant5/1 -> Sum3/1, GreaterThan6/2, COMM Task - Set_Values/1(Time Mark)
  Constant13/1 -> GreaterThan/2, Sum4/1, COMP Task - Sync bc1 check/2(TM_COMM), COMM Task - Sync bc 1/1(Time Mark)
  GreaterThan/1 -> AND/1
  GreaterThan1/1 -> AND/2
  NOT4/1 -> AND17/2
  Data Store Read6/1 -> NOT2/1
  AND2/1 -> AND19/1
  AND17/1 -> COMM Task - Sync bc 1/Enable
  Data Store Read11/1 -> NOT4/1
  AND1/1 -> AND18/1
  AND18/1 -> COMP Task - Sync bc1 check/Enable
  AND3/1 -> COMM Task - Set_Values/Enable
  GreaterThan4/1 -> AND2/1
  Data Store Read7/1 -> NOT5/1
  Constant9/1 -> Sum5/2
  NOT2/1 -> AND18/2
  AND4/1 -> COMP Task - Reset Board/Enable
  AND19/1 -> COMP Task - Update LT/Enable
  COMM Task - Sync bc 1/4(Receive CAN2) -> [receive_CAN2_Sync_bc1_TAG]
  COMM Task - Sync bc 1/2(Receive CAN1) -> [receive_CAN1_Sync_bc1_TAG]
  COMM Task - Sync bc 1/1(Send CAN1) -> [send_CAN1_Sync_bc1_TAG]
  Constant1/1 -> Sum4/2
  [receive_CAN2_Set_Values_bc1_TAG] -> OR2/2
  [receive_CAN2_Sync_bc1_TAG] -> OR2/1
  [receive_CAN1_Set_Values_bc1_TAG] -> OR3/2
  [receive_CAN1_Sync_bc1_TAG] -> OR3/1
  [send_CAN2_Set_Values_bc1_TAG] -> OR4/2
  [send_CAN2_Sync_bc1_TAG] -> OR4/1
  [send_CAN1_Set_Values_bc1_TAG] -> OR1/2
  [send_CAN1_Sync_bc1_TAG] -> OR1/1
  OR3/1 -> Receive_Message_CAN1/1
  OR4/1 -> Send_Message_CAN2/1
  OR2/1 -> Receive_Message_CAN2/1
  OR1/1 -> Send_Message_CAN1/1
  Constant8/1 -> COMP Task - Rx_Set_Values_Check/1(Time_Mark), Sum6/1, GreaterThan10/2
  GreaterThan10/1 -> AND5/1
  Data Store Read1/1 -> GreaterThan1/1, GreaterThan/1, GreaterThan3/1, GreaterThan2/1, GreaterThan5/1, GreaterThan4/1, GreaterThan7/1, GreaterThan6/1, GreaterThan35/1, GreaterThan34/1, GreaterThan9/1, GreaterThan8/1, GreaterThan11/1, GreaterThan10/1
  GreaterThan11/1 -> AND5/2
  Constant10/1 -> Sum6/2
  Sum6/1 -> GreaterThan11/2
  AND5/1 -> COMP Task - Rx_Set_Values_Check/Enable
  Constant11/1 -> COMP Task - Update LT/2(Time_Mark_2)
  Constant12/1 -> COMP Task - Reset Board/2(Time_Mark_2)

== system HANcoder_E407_TTA_Group2_REMOTE_72/HANcoder STM32 Target - E407-STM32 algorithm/TTA CAN System/TTA System/Matrix Cycle Manager/Input Generator Matrix Cycle/msg_count_DEBUG observer ==
  Data Store Read24 : DataStoreRead  DataStoreName=msg_count_DEBUG
  Terminator : Terminator
  wires:
  Data Store Read24/1 -> Terminator/1  "msg_count_DEBUG_ing_s"

== system HANcoder_E407_TTA_Group2_REMOTE_72/HANcoder STM32 Target - E407-STM32 algorithm/TTA CAN System/TTA System/Matrix Cycle Manager/Vehicle Emulator Matrix Cycle/Matrix_Cycle_Observation_DEBUG ==
  Data Store Read : DataStoreRead  DataStoreName=Master_ID
  Data Store Read1 : DataStoreRead  DataStoreName=Role_ID
  Data Store Read10 : DataStoreRead  DataStoreName=BC1_Sync_processed
  Data Store Read2 : DataStoreRead  DataStoreName=BC0_Sync_processed
  Data Store Read3 : DataStoreRead  DataStoreName=Sync_bc1_missed_counter
  Data Store Read4 : DataStoreRead  DataStoreName=Sync_bc0_missed_counter
  Data Store Read5 : DataStoreRead  DataStoreName=OutController_missed_counter
  Terminator{,1..5,12} (7 alike) : Terminator
  wires:
  Data Store Read1/1 -> Terminator/1  "Role_ID_vem_s"
  Data Store Read10/1 -> Terminator12/1  "BC1_sync_processed_vem__s"
  Data Store Read2/1 -> Terminator2/1  "BC0_sync_processed_vem__s"
  Data Store Read/1 -> Terminator1/1  "Master_ID_vem_s"
  Data Store Read5/1 -> Terminator5/1  "outcont_miss_counter_vem"
  Data Store Read3/1 -> Terminator4/1  "sync_bc1_miss_counter_vem"
  Data Store Read4/1 -> Terminator3/1  "sync_bc0_miss_counter_vem"

== system HANcoder_E407_TTA_Group2_REMOTE_72/HANcoder STM32 Target - E407-STM32 algorithm/TTA CAN System/TTA System/Matrix Cycle Manager/Vehicle Emulator Matrix Cycle/msg_count_DEBUG observer ==
  Data Store Read24 : DataStoreRead  DataStoreName=msg_count_DEBUG
  Terminator : Terminator
  wires:
  Data Store Read24/1 -> Terminator/1  "msg_count_DEBUG_vem_s"

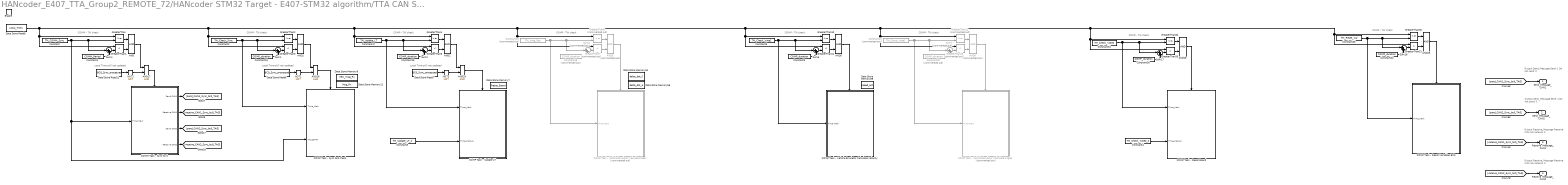
== system HANcoder_E407_TTA_Group2_REMOTE_72/HANcoder STM32 Target - E407-STM32 algorithm/TTA CAN System/TTA System/Matrix Cycle Manager/Vehicle Emulator Matrix Cycle/vehicle emulator basic cycle 0 ==
  note: Output Send_Message
      | Send: 1
      | Do not send: 0
  note: Output Receive_Message
      | Receive: 1
      | Do not receive: 0
  note: Output Send_Message
      | Send: 1
      | Do not send: 0
  note: Output Receive_Message
      | Receive: 1
      | Do not receive: 0
  note: COMM - TW check
  note: COMP - TW check
  note: COMP - TW check
  note: COMP - TW check
  note: COMP - TW check
  note: COMP - TW check
  note: COMP - TW check
  note: COMP - TW check
  note: Local Time still not updated
  note: Local Time still not updated
  note: Local Time still not updated
  Enable : EnablePort  PropagateVarSize=During execution
  AND{,1..2,5,15..19} (9 alike) : Logic  IconShape=distinctive  AllPortsSameDT=off  OutDataTypeStr=boolean
  AND3 : Logic  Commented=on  IconShape=distinctive  AllPortsSameDT=off  OutDataTypeStr=boolean
  AND6 : Logic  Commented=on  IconShape=distinctive  AllPortsSameDT=off  OutDataTypeStr=boolean
  COMM Task - Sync bc 0 : Subsystem
  COMP Task - Reset Board : Subsystem
  COMP Task - Reset Variables BC0 : Subsystem
  COMP Task - Sync bc0 check : Subsystem
  COMP Task - Update LT : Subsystem
  COMP Task - Vehicle Emulator Calculate Angles : Subsystem  Commented=on
  COMP Task - Vehicle Emulator Calculate Steer : Subsystem  Commented=on
  COMP Task - Vehicle Emulator Calculate Velocity : Subsystem
  Constant : Constant  Value=TM_COMM_Sync
  Constant1 : Constant  Value=COMM_Period
  Constant{5,15..16,24,30} (5 alike) : Constant  Value=COMP_duration
  Constant17 : Constant  Value=TM_Update_LT
  Constant18 : Constant  Commented=on  Value=COMP_duration
  Constant19 : Constant  Commented=on  Value=TM_Vote_Dec
  Constant2 : Constant  Value=TM_Check_Sync
  Constant20 : Constant  Commented=on  Value=COMP_duration
  Constant21 : Constant  Commented=on  Value=TM_Count_Vote1
  Constant25 : Constant  Value=TM_Reset_Var
  Constant3 : Constant  Value=TM_Update_LT_2
  Constant31 : Constant  Value=TM_Check_Vote2
  Constant4 : Constant  Value=TM_Check_Vote2_2
  Constant6 : Constant  Value=TM_Check_Vote1
  Data Store Memory11 : DataStoreMemory  DataStoreName=Msg_Rx  ReadBeforeWriteMsg=warning  WriteAfterWriteMsg=warning  WriteAfterReadMsg=warning  ShowAdditionalParam=off  OutDataTypeStr=Bus: msg_buffer_type
  Data Store Memory54 : DataStoreMemory  DataStoreName=delta_dot_f  ReadBeforeWriteMsg=warning  WriteAfterWriteMsg=warning  WriteAfterReadMsg=warning  ShowAdditionalParam=off
  Data Store Memory56 : DataStoreMemory  DataStoreName=delta_dot_a  ReadBeforeWriteMsg=warning  WriteAfterWriteMsg=warning  WriteAfterReadMsg=warning  ShowAdditionalParam=off
  Data Store Memory59 : DataStoreMemory  DataStoreName=speed_act  ReadBeforeWriteMsg=warning  WriteAfterWriteMsg=warning  WriteAfterReadMsg=warning  ShowAdditionalParam=off
  Data Store Memory7 : DataStoreMemory  DataStoreName=Reset_Board  ReadBeforeWriteMsg=warning  WriteAfterWriteMsg=warning  WriteAfterReadMsg=warning  ShowAdditionalParam=off  OutDataTypeStr=boolean
  Data Store Memory8 : DataStoreMemory  DataStoreName=new_msg_Rx  ReadBeforeWriteMsg=warning  WriteAfterWriteMsg=warning  WriteAfterReadMsg=warning  ShowAdditionalParam=off
  Data Store Read11 : DataStoreRead  DataStoreName=BC0_Sync_processed
  Data Store Read6 : DataStoreRead  DataStoreName=BC0_Sync_processed
  Data Store Read7 : DataStoreRead  DataStoreName=BC0_Sync_processed
  Data Store Read8 : DataStoreRead  DataStoreName=Local_Ticks
  GreaterThan{,2,4,10,30,32} (6 alike) : RelationalOperator  OutDataTypeStr=boolean  RndMeth=Simplest
  GreaterThan{1,3,5,11,31,33} (6 alike) : RelationalOperator  Operator=<  OutDataTypeStr=boolean  RndMeth=Simplest
  GreaterThan12 : RelationalOperator  Commented=on  OutDataTypeStr=boolean  RndMeth=Simplest
  GreaterThan13 : RelationalOperator  Commented=on  Operator=<  OutDataTypeStr=boolean  RndMeth=Simplest
  GreaterThan6 : RelationalOperator  Commented=on  OutDataTypeStr=boolean  RndMeth=Simplest
  GreaterThan7 : RelationalOperator  Commented=on  Operator=<  OutDataTypeStr=boolean  RndMeth=Simplest
  NOT1 : Logic  Operator=NOT  IconShape=distinctive  AllPortsSameDT=off  OutDataTypeStr=boolean
  NOT2 : Logic  Operator=NOT  IconShape=distinctive  AllPortsSameDT=off  OutDataTypeStr=boolean
  NOT3 : Logic  Operator=NOT  IconShape=distinctive  AllPortsSameDT=off  OutDataTypeStr=boolean
  Sum{1..2,4,6,16..17} (6 alike) : Sum  Inputs=|++
  Sum3 : Sum  Commented=on  Inputs=|++
  Sum7 : Sum  Commented=on  Inputs=|++
  Send_Message_CAN1 : Outport  OutputWhenDisabled=reset  InitialOutput=0
  Send_Message_CAN2 : Outport  Port=2  OutputWhenDisabled=reset  InitialOutput=0
  Receive_Message_CAN1 : Outport  Port=3  OutputWhenDisabled=reset  InitialOutput=0
  Receive_Message_CAN2 : Outport  Port=4  OutputWhenDisabled=reset  InitialOutput=0
  wires:
  COMM Task - Sync bc 0/1(Send CAN1) -> [send_CAN1_Sync_bc0_TAG]
  COMM Task - Sync bc 0/2(Receive CAN1) -> [receive_CAN1_Sync_bc0_TAG]
  COMM Task - Sync bc 0/3(Send CAN2) -> [send_CAN2_Sync_bc0_TAG]
  COMM Task - Sync bc 0/4(Receive CAN2) -> [receive_CAN2_Sync_bc0_TAG]
  Constant1/1 -> Sum4/2
  Constant/1 -> COMP Task - Sync bc0 check/2(TM_COMM), COMM Task - Sync bc 0/1(Time Mark), Sum4/1, GreaterThan/2
  Sum4/1 -> GreaterThan1/2
  GreaterThan/1 -> AND/1
  GreaterThan1/1 -> AND/2
  AND/1 -> AND17/1
  GreaterThan3/1 -> AND1/2
  GreaterThan2/1 -> AND1/1
  Sum1/1 -> GreaterThan3/2
  Constant2/1 -> COMP Task - Sync bc0 check/1(Time_Mark), GreaterThan2/2, Sum1/1
  Constant15/1 -> Sum1/2
  Constant16/1 -> Sum2/2
  Constant17/1 -> COMP Task - Update LT/1(Time_Mark), Sum2/1, GreaterThan4/2
  Sum2/1 -> GreaterThan5/2
  GreaterThan4/1 -> AND2/1
  GreaterThan5/1 -> AND2/2
  AND3/1 -> COMP Task - Vehicle Emulator Calculate Steer/Enable
  GreaterThan7/1 -> AND3/2
  GreaterThan6/1 -> AND3/1
  Sum3/1 -> GreaterThan7/2
  Constant19/1 -> COMP Task - Vehicle Emulator Calculate Steer/1(Time Mark), GreaterThan6/2, Sum3/1
  Constant18/1 -> Sum3/2
  GreaterThan11/1 -> AND5/2
  Sum6/1 -> GreaterThan11/2
  GreaterThan10/1 -> AND5/1
  Constant5/1 -> Sum6/2
  Constant6/1 -> COMP Task - Vehicle Emulator Calculate Velocity/1(Time Mark), GreaterThan10/2, Sum6/1
  AND5/1 -> COMP Task - Vehicle Emulator Calculate Velocity/Enable
  AND6/1 -> COMP Task - Vehicle Emulator Calculate Angles/Enable
  Constant21/1 -> COMP Task - Vehicle Emulator Calculate Angles/1(Time Mark), Sum7/1, GreaterThan12/2
  Constant20/1 -> Sum7/2
  GreaterThan12/1 -> AND6/1
  Sum7/1 -> GreaterThan13/2
  GreaterThan13/1 -> AND6/2
  GreaterThan31/1 -> AND15/2
  Sum16/1 -> GreaterThan31/2
  GreaterThan30/1 -> AND15/1
  Constant24/1 -> Sum16/2
  Constant25/1 -> COMP Task - Reset Variables BC0/1(Time_Mark), GreaterThan30/2, Sum16/1
  AND15/1 -> COMP Task - Reset Variables BC0/Enable
  Data Store Read8/1 -> GreaterThan31/1, GreaterThan30/1, GreaterThan32/1, GreaterThan33/1, GreaterThan12/1, GreaterThan13/1, GreaterThan11/1, GreaterThan10/1, GreaterThan6/1, GreaterThan7/1, GreaterThan4/1, GreaterThan5/1, GreaterThan2/1, GreaterThan3/1, GreaterThan/1, GreaterThan1/1
  AND16/1 -> COMP Task - Reset Board/Enable
  Constant31/1 -> COMP Task - Reset Board/1(Time_Mark), Sum17/1, GreaterThan32/2
  Constant30/1 -> Sum17/2
  GreaterThan32/1 -> AND16/1
  Sum17/1 -> GreaterThan33/2
  GreaterThan33/1 -> AND16/2
  Data Store Read11/1 -> NOT2/1
  NOT2/1 -> AND17/2
  AND17/1 -> COMM Task - Sync bc 0/Enable
  Data Store Read6/1 -> NOT1/1
  NOT1/1 -> AND18/2
  AND1/1 -> AND18/1
  AND18/1 -> COMP Task - Sync bc0 check/Enable
  Data Store Read7/1 -> NOT3/1
  NOT3/1 -> AND19/2
  AND2/1 -> AND19/1
  AND19/1 -> COMP Task - Update LT/Enable
  [send_CAN2_Sync_bc0_TAG] -> Send_Message_CAN2/1
  [receive_CAN1_Sync_bc0_TAG] -> Receive_Message_CAN1/1
  [receive_CAN2_Sync_bc0_TAG] -> Receive_Message_CAN2/1
  [send_CAN1_Sync_bc0_TAG] -> Send_Message_CAN1/1
  Constant3/1 -> COMP Task - Update LT/2(Time_Mark_2)
  Constant4/1 -> COMP Task - Reset Board/2(Time_Mark_2)
